simulink model "ddc_model"  (R2023b)
settings: Solver=VariableStepDiscrete  StartTime=0.0  StopTime=DDC_LINEUP_param.endTime  RelTol=1e-3  EnableMultiTasking=on
PreLoadFcn:
  | % Run the setup script when the model is opened
  | setup_ddc_model;
InitFcn:
  | % Run the setup script again just before the
  | % model is run, so that any updates made
  | % after opening are applied.
  | 
  | setup_ddc_model;
StopFcn:
  | ddc_output_analysis;
values from neighbouring files (symbols this model uses):
  DDC_CM_multiplication_factor = 1    [setup_ddc_model.m]
  DDC_CM_NCO1_phase = [0 0 0 0]*2^DDC_LINEUP_param.Complex_NCO1.accum_bit_width    [setup_ddc_model.m]
  DDC_CM_NCO_sync = [0 0 0 0]    [setup_ddc_model.m]
  DDC_CM_number_of_bits_to_shift_left = 0    [setup_ddc_model.m]
undefined symbols (not defined in the file or in its folder): AdvDSPBChannelOutDisplay, COMPLEX_MIXER, DDC_LINEUP_param, dpoly, dspba_ChannelInVis, dspba_ChannelOutVis, dspba_internal_get_channel_ports, evalAionMaskParam, latency, lddc, lddc_lib, mixer_lib, primtype, value
libraries: DSPBAPrim x43, DSPBABase x15, simulink x10, DSPBAFilters x6, DSPBAModelBus x3, DSPBAWaveformSynth x2
(part 2 of 2)

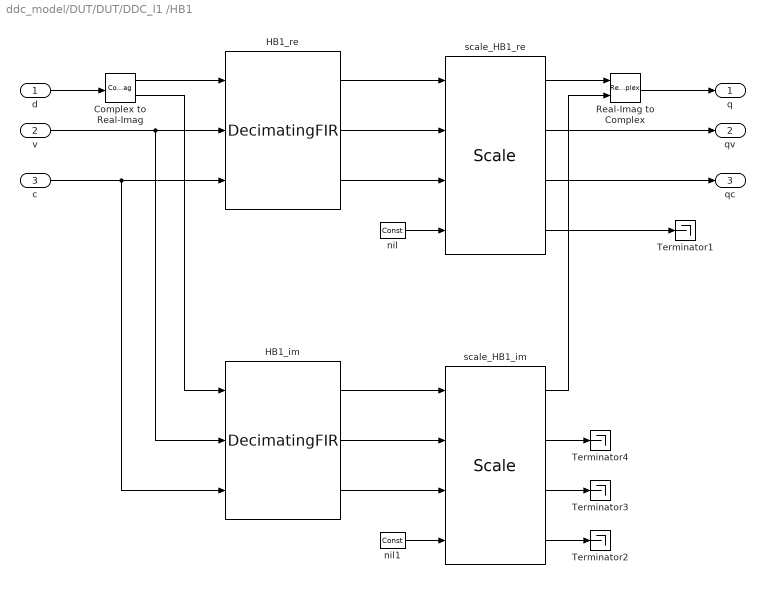
== system ddc_model/DUT/DUT/DDC_l1 /HB1 ==
  d : Inport
  v : Inport  Port=2
  c : Inport  Port=3
  Complex to Real-Imag : ComplexToRealImag
  HB1_im : DSPBAFilters/DecimatingFIR  nInputRate=DDC_LINEUP_param.HB_filt1.SampleRate  decim=DDC_LINEUP_param.HB_filt1.Decimation  nchan=DDC_LINEUP_param.HB_filt1.ChanCount  symmetry=Symmetrical  coef=DDC_LINEUP_param.HB_filt1.coeffs  addr=DDC_LINEUP_param.HB_filter6_3.base_addr  rwmode=Constant  nband=Half Band  exposebus=off  latency=17  version=20090407  recon=off  MM=[0,1,2,3,4,5,6,7,8,9,10,11,12,13,14,15]  resetrezero=off  sharecoef=auto  simulationMode=Standard
  HB1_re : DSPBAFilters/DecimatingFIR  nInputRate=DDC_LINEUP_param.HB_filt1.SampleRate  decim=DDC_LINEUP_param.HB_filt1.Decimation  nchan=DDC_LINEUP_param.HB_filt1.ChanCount  symmetry=Symmetrical  coef=DDC_LINEUP_param.HB_filt1.coeffs  addr=DDC_LINEUP_param.HB_filter6_3.base_addr  rwmode=Constant  nband=Half Band  exposebus=off  latency=17  version=20090407  recon=off  MM=[0,1,2,3,4,5,6,7,8,9,10,11,12,13,14,15]  resetrezero=off  sharecoef=auto  simulationMode=Standard
  Real-Imag to Complex : RealImagToComplex
  Terminator{1..4} (4 alike) : Terminator
  nil : DSPBAPrim/Const  primtype=const  nInputs=0  nOutputs=1  omode=Inherit via internal rule  otype=sfix(16)  scale=2^-15  rndmethod=Unbiased  factor=1  satmethod=Symmetric  shift_vec=[0 1 2 -1]  value=0  inPortNames=['+'; '+';]  outPortNames=[' ']  dspbaimage=dspba_prim.svg  text=fprintf('%s', num2str(value));  style=Optimised  visibilities=8 + 1024  floatPrecision=float32_m23  warnSaturation=on  version=20211007  SampleTime=inf
  nil1 : DSPBAPrim/Const  primtype=const  nInputs=0  nOutputs=1  omode=Inherit via internal rule  otype=sfix(16)  scale=2^-15  rndmethod=Unbiased  factor=1  satmethod=Symmetric  shift_vec=[0 1 2 -1]  value=0  inPortNames=['+'; '+';]  outPortNames=[' ']  dspbaimage=dspba_prim.svg  text=fprintf('%s', num2str(value));  style=Optimised  visibilities=8 + 1024  floatPrecision=float32_m23  warnSaturation=on  version=20211007  SampleTime=inf
  scale_HB1_im : DSPBABase/Scale  otype=sfix(DDC_LINEUP_param.output_word_length)  scale=2^-DDC_LINEUP_param.output_fraction_length  rndmethod=Biased  factor=1  satmethod=None  shift_vec=0  latency=2  simulationMode=Use Global Value  version=20130807
  scale_HB1_re : DSPBABase/Scale  otype=sfix(DDC_LINEUP_param.output_word_length)  scale=2^-DDC_LINEUP_param.output_fraction_length  rndmethod=Biased  factor=1  satmethod=None  shift_vec=0  latency=2  simulationMode=Use Global Value  version=20130807
  q : Outport
  qv : Outport  Port=2
  qc : Outport  Port=3
  wires:
  scale_HB1_re/1 -> Real-Imag to Complex/1
  HB1_re/3 -> scale_HB1_re/3
  c/1 -> HB1_im/3, HB1_re/3
  scale_HB1_re/3 -> qc/1
  scale_HB1_re/2 -> qv/1
  HB1_re/2 -> scale_HB1_re/2
  v/1 -> HB1_im/2, HB1_re/2
  nil1/1 -> scale_HB1_im/4
  scale_HB1_re/4 -> Terminator1/1
  HB1_re/1 -> scale_HB1_re/1
  Complex to Real-Imag/1 -> HB1_re/1
  nil/1 -> scale_HB1_re/4
  d/1 -> Complex to Real-Imag/1
  scale_HB1_im/4 -> Terminator2/1
  HB1_im/1 -> scale_HB1_im/1
  scale_HB1_im/1 -> Real-Imag to Complex/2
  scale_HB1_im/2 -> Terminator4/1
  Complex to Real-Imag/2 -> HB1_im/1
  HB1_im/2 -> scale_HB1_im/2
  scale_HB1_im/3 -> Terminator3/1
  Real-Imag to Complex/1 -> q/1
  HB1_im/3 -> scale_HB1_im/3

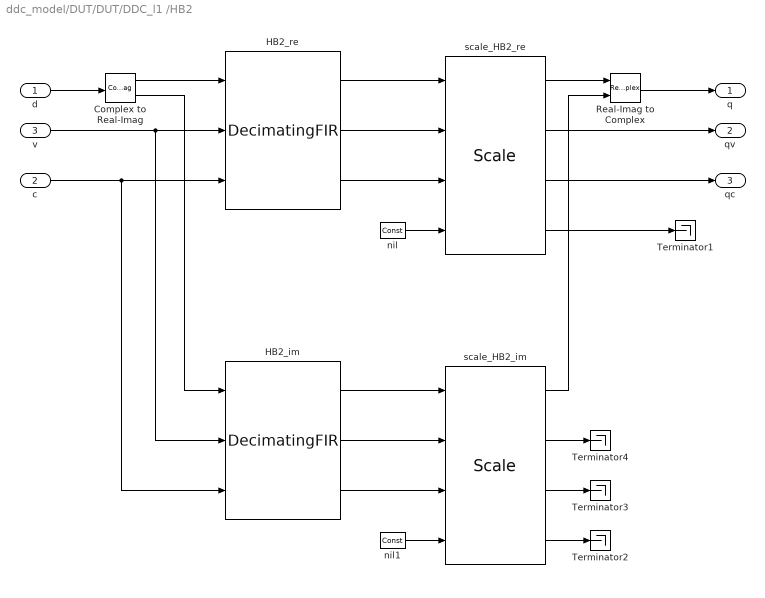
== system ddc_model/DUT/DUT/DDC_l1 /HB2 ==
  d : Inport
  c : Inport  Port=2
  v : Inport  Port=3
  Complex to Real-Imag : ComplexToRealImag
  HB2_im : DSPBAFilters/DecimatingFIR  nInputRate=DDC_LINEUP_param.HB_filt2.SampleRate  decim=DDC_LINEUP_param.HB_filt2.Decimation  nchan=DDC_LINEUP_param.HB_filt2.ChanCount  symmetry=Symmetrical  coef=DDC_LINEUP_param.HB_filt2.coeffs  addr=DDC_LINEUP_param.HB_filter6_3.base_addr  rwmode=Constant  nband=Half Band  exposebus=off  latency=16  version=20090407  recon=off  MM=[0,1,2,3,4,5,6,7,8,9,10,11,12,13,14,15]  resetrezero=off  sharecoef=auto  simulationMode=Standard
  HB2_re : DSPBAFilters/DecimatingFIR  nInputRate=DDC_LINEUP_param.HB_filt2.SampleRate  decim=DDC_LINEUP_param.HB_filt2.Decimation  nchan=DDC_LINEUP_param.HB_filt2.ChanCount  symmetry=Symmetrical  coef=DDC_LINEUP_param.HB_filt2.coeffs  addr=DDC_LINEUP_param.HB_filter6_3.base_addr  rwmode=Constant  nband=Half Band  exposebus=off  latency=16  version=20090407  recon=off  MM=[0,1,2,3,4,5,6,7,8,9,10,11,12,13,14,15]  resetrezero=off  sharecoef=auto  simulationMode=Standard
  Real-Imag to Complex : RealImagToComplex
  Terminator{1..4} (4 alike) : Terminator
  nil : DSPBAPrim/Const  primtype=const  nInputs=0  nOutputs=1  omode=Inherit via internal rule  otype=sfix(16)  scale=2^-15  rndmethod=Unbiased  factor=1  satmethod=Symmetric  shift_vec=[0 1 2 -1]  value=0  inPortNames=['+'; '+';]  outPortNames=[' ']  dspbaimage=dspba_prim.svg  text=fprintf('%s', num2str(value));  style=Optimised  visibilities=8 + 1024  floatPrecision=float32_m23  warnSaturation=on  version=20211007  SampleTime=inf
  nil1 : DSPBAPrim/Const  primtype=const  nInputs=0  nOutputs=1  omode=Inherit via internal rule  otype=sfix(16)  scale=2^-15  rndmethod=Unbiased  factor=1  satmethod=Symmetric  shift_vec=[0 1 2 -1]  value=0  inPortNames=['+'; '+';]  outPortNames=[' ']  dspbaimage=dspba_prim.svg  text=fprintf('%s', num2str(value));  style=Optimised  visibilities=8 + 1024  floatPrecision=float32_m23  warnSaturation=on  version=20211007  SampleTime=inf
  scale_HB2_im : DSPBABase/Scale  otype=sfix(DDC_LINEUP_param.output_word_length)  scale=2^-DDC_LINEUP_param.output_fraction_length  rndmethod=Biased  factor=1  satmethod=None  shift_vec=0  latency=2  simulationMode=Use Global Value  version=20130807
  scale_HB2_re : DSPBABase/Scale  otype=sfix(DDC_LINEUP_param.output_word_length)  scale=2^-DDC_LINEUP_param.output_fraction_length  rndmethod=Biased  factor=1  satmethod=None  shift_vec=0  latency=2  simulationMode=Use Global Value  version=20130807
  q : Outport
  qv : Outport  Port=2
  qc : Outport  Port=3
  wires:
  HB2_im/3 -> scale_HB2_im/3
  Real-Imag to Complex/1 -> q/1
  scale_HB2_im/3 -> Terminator3/1
  HB2_im/2 -> scale_HB2_im/2
  Complex to Real-Imag/2 -> HB2_im/1
  scale_HB2_im/2 -> Terminator4/1
  scale_HB2_im/1 -> Real-Imag to Complex/2
  HB2_im/1 -> scale_HB2_im/1
  scale_HB2_im/4 -> Terminator2/1
  d/1 -> Complex to Real-Imag/1
  nil/1 -> scale_HB2_re/4
  Complex to Real-Imag/1 -> HB2_re/1
  HB2_re/1 -> scale_HB2_re/1
  scale_HB2_re/4 -> Terminator1/1
  nil1/1 -> scale_HB2_im/4
  v/1 -> HB2_im/2, HB2_re/2
  HB2_re/2 -> scale_HB2_re/2
  scale_HB2_re/2 -> qv/1
  scale_HB2_re/3 -> qc/1
  c/1 -> HB2_im/3, HB2_re/3
  HB2_re/3 -> scale_HB2_re/3
  scale_HB2_re/1 -> Real-Imag to Complex/1

== system ddc_model/DUT/DUT/DDC_l1 /routing_reg_hb62hb7 ==
  d : Inport
  dv : Inport  Port=2
  dc : Inport  Port=3
  ChannelIn : DSPBAPrim/ChannelIn  primtype=channelin  nInputs=dspba_internal_get_channel_ports(gcb)  nOutputs=dspba_internal_get_channel_ports(gcb)  omode=Inherit via internal rule  otype=sfix(16)  scale=2^-15  rndmethod=Unbiased  factor=1  satmethod=Symmetric  shift_vec=[0 1 2 -1]  value=1  inPortNames=['v'; 'c'; '0'; '1'; '2'; '3'; '4'; '5'; '6'; '7'; '8'; '9'; 'A'; 'B'; 'D'; 'E'; 'F'; 'G'; 'H'; 'I'; 'J'; 'K'; 'L'; 'M'; 'N'; 'O'; 'P'; 'Q'; 'R'; 'S'; 'T'; 'U'; 'W'; 'X'; 'Y'; 'Z']  outPortNames=['v'; 'c'; '0'; '1'; '2'; '3'; '4'; '5'; '6'; '7'; '8'; '9'; 'A'; 'B'; 'D'; 'E'; 'F'; 'G'; 'H'; 'I'; 'J'; 'K'; 'L'; 'M'; 'N'; 'O'; 'P'; 'Q'; 'R'; 'S'; 'T'; 'U'; 'W'; 'X'; 'Y'; 'Z']  dspbaimage=dspba_prim_channel_tall.svg  text=fprintf('In');  style=Optimised  dataSignals=1  foldingEnabled=off  channels=1  sampleRate=200  packetBeginPresent=off  packetBeginEnabled=off  visibilities=dspba_ChannelInVis(gcb)  scheduleOrigin=on  version=20211214
  ChannelOut : DSPBAPrim/ChannelOut  primtype=channelout  nInputs=dspba_internal_get_channel_ports(gcb)  nOutputs=dspba_internal_get_channel_ports(gcb)  omode=Inherit via internal rule  otype=sfix(16)  scale=2^-15  rndmethod=Unbiased  factor=1  satmethod=Symmetric  shift_vec=[0 1 2 -1]  value=1  inPortNames=['v'; 'c'; '0'; '1'; '2'; '3'; '4'; '5'; '6'; '7'; '8'; '9'; 'A'; 'B'; 'D'; 'E'; 'F'; 'G'; 'H'; 'I'; 'J'; 'K'; 'L'; 'M'; 'N'; 'O'; 'P'; 'Q'; 'R'; 'S'; 'T'; 'U'; 'W'; 'X'; 'Y'; 'Z']  outPortNames=['v'; 'c'; '0'; '1'; '2'; '3'; '4'; '5'; '6'; '7'; '8'; '9'; 'A'; 'B'; 'D'; 'E'; 'F'; 'G'; 'H'; 'I'; 'J'; 'K'; 'L'; 'M'; 'N'; 'O'; 'P'; 'Q'; 'R'; 'S'; 'T'; 'U'; 'W'; 'X'; 'Y'; 'Z']  dspbaimage=dspba_prim_channel_tall.svg  text=fprintf('Out%s', AdvDSPBChannelOutDisplay(latency));  style=Optimised  dataSignals=1  foldingEnabled=off  channels=1  sampleRate=200  packetBeginPresent=off  packetBeginEnabled=off  visibilities=dspba_ChannelOutVis(gcb)  latency=3  version=20211214
  SynthesisInfo : DSPBAPrim/SynthesisInfo  primtype=synthinfo  nInputs=0  nOutputs=0  omode=Inherit via internal rule  otype=sfix(16)  scale=2^-15  rndmethod=Truncate  factor=1  satmethod=Symmetric  shift_vec=[0 1 2 -1]  value=99  inPortNames=[' '; ' ';]  outPortNames=[' ']  dspbaimage=dspba_prim_ctrl.jpg  text=fprintf('Style=%s', style);  style=Scheduled  visibilities=2^17+2^18+2^19+2^20  constraintPair=Channel-In to Channel-Out  constraintRelation=>  constraintLimit=2  modelRefSign=+  modelRef=''  showSchedule=off  simulationMode=Use Global Value  resetMinimization=Conditional - On for ChannelIn/Out only  version=20220106
  q0 : Outport
  qv : Outport  Port=2
  qc : Outport  Port=3
  wires:
  dv/1 -> ChannelIn/1
  d/1 -> ChannelIn/3
  ChannelIn/1 -> ChannelOut/1
  ChannelIn/2 -> ChannelOut/2
  ChannelIn/3 -> ChannelOut/3
  ChannelOut/3 -> q0/1
  ChannelOut/1 -> qv/1
  ChannelOut/2 -> qc/1
  dc/1 -> ChannelIn/2

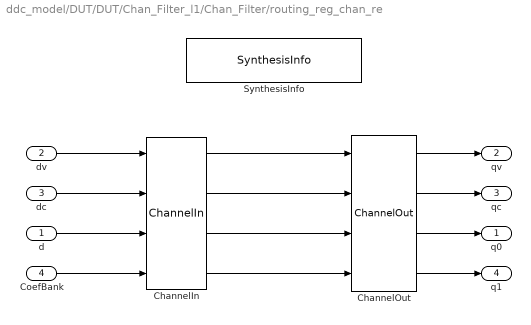
== system ddc_model/DUT/DUT/Chan_Filter_l1/Chan_Filter/routing_reg_chan_re ==
  d : Inport
  dv : Inport  Port=2
  dc : Inport  Port=3
  CoefBank : Inport  Port=4
  ChannelIn : DSPBAPrim/ChannelIn  primtype=channelin  nInputs=dspba_internal_get_channel_ports(gcb)  nOutputs=dspba_internal_get_channel_ports(gcb)  omode=Inherit via internal rule  otype=sfix(16)  scale=2^-15  rndmethod=Unbiased  factor=1  satmethod=Symmetric  shift_vec=[0 1 2 -1]  value=2  inPortNames=['v'; 'c'; '0'; '1'; '2'; '3'; '4'; '5'; '6'; '7'; '8'; '9'; 'A'; 'B'; 'D'; 'E'; 'F'; 'G'; 'H'; 'I'; 'J'; 'K'; 'L'; 'M'; 'N'; 'O'; 'P'; 'Q'; 'R'; 'S'; 'T'; 'U'; 'W'; 'X'; 'Y'; 'Z']  outPortNames=['v'; 'c'; '0'; '1'; '2'; '3'; '4'; '5'; '6'; '7'; '8'; '9'; 'A'; 'B'; 'D'; 'E'; 'F'; 'G'; 'H'; 'I'; 'J'; 'K'; 'L'; 'M'; 'N'; 'O'; 'P'; 'Q'; 'R'; 'S'; 'T'; 'U'; 'W'; 'X'; 'Y'; 'Z']  dspbaimage=dspba_prim_channel_tall.svg  text=fprintf('In');  style=Optimised  dataSignals=2  foldingEnabled=off  channels=1  sampleRate=200  packetBeginPresent=off  packetBeginEnabled=off  visibilities=dspba_ChannelInVis(gcb)  scheduleOrigin=on  version=20211214
  ChannelOut : DSPBAPrim/ChannelOut  primtype=channelout  nInputs=dspba_internal_get_channel_ports(gcb)  nOutputs=dspba_internal_get_channel_ports(gcb)  omode=Inherit via internal rule  otype=sfix(16)  scale=2^-15  rndmethod=Unbiased  factor=1  satmethod=Symmetric  shift_vec=[0 1 2 -1]  value=2  inPortNames=['v'; 'c'; '0'; '1'; '2'; '3'; '4'; '5'; '6'; '7'; '8'; '9'; 'A'; 'B'; 'D'; 'E'; 'F'; 'G'; 'H'; 'I'; 'J'; 'K'; 'L'; 'M'; 'N'; 'O'; 'P'; 'Q'; 'R'; 'S'; 'T'; 'U'; 'W'; 'X'; 'Y'; 'Z']  outPortNames=['v'; 'c'; '0'; '1'; '2'; '3'; '4'; '5'; '6'; '7'; '8'; '9'; 'A'; 'B'; 'D'; 'E'; 'F'; 'G'; 'H'; 'I'; 'J'; 'K'; 'L'; 'M'; 'N'; 'O'; 'P'; 'Q'; 'R'; 'S'; 'T'; 'U'; 'W'; 'X'; 'Y'; 'Z']  dspbaimage=dspba_prim_channel_tall.svg  text=fprintf('Out%s', AdvDSPBChannelOutDisplay(latency));  style=Optimised  dataSignals=2  foldingEnabled=off  channels=1  sampleRate=200  packetBeginPresent=off  packetBeginEnabled=off  visibilities=dspba_ChannelOutVis(gcb)  latency=3  version=20211214
  SynthesisInfo : DSPBAPrim/SynthesisInfo  primtype=synthinfo  nInputs=0  nOutputs=0  omode=Inherit via internal rule  otype=sfix(16)  scale=2^-15  rndmethod=Truncate  factor=1  satmethod=Symmetric  shift_vec=[0 1 2 -1]  value=99  inPortNames=[' '; ' ';]  outPortNames=[' ']  dspbaimage=dspba_prim_ctrl.jpg  text=fprintf('Style=%s', style);  style=Scheduled  visibilities=2^17+2^18+2^19+2^20  constraintPair=Channel-In to Channel-Out  constraintRelation=>  constraintLimit=2  modelRefSign=+  modelRef=''  showSchedule=off  simulationMode=Use Global Value  resetMinimization=Conditional - On for ChannelIn/Out only  version=20220106
  q0 : Outport
  qv : Outport  Port=2
  qc : Outport  Port=3
  q1 : Outport  Port=4
  wires:
  dv/1 -> ChannelIn/1
  d/1 -> ChannelIn/3
  ChannelIn/1 -> ChannelOut/1
  ChannelIn/2 -> ChannelOut/2
  ChannelIn/3 -> ChannelOut/3
  ChannelOut/3 -> q0/1
  ChannelOut/1 -> qv/1
  ChannelOut/2 -> qc/1
  dc/1 -> ChannelIn/2
  ChannelIn/4 -> ChannelOut/4
  CoefBank/1 -> ChannelIn/4
  ChannelOut/4 -> q1/1

== system ddc_model/DUT/DUT/Chan_Filter_l1/Chan_Filter/routing_reg_chan_re1 ==
  d : Inport
  dv : Inport  Port=2
  dc : Inport  Port=3
  CoefBank : Inport  Port=4
  ChannelIn : DSPBAPrim/ChannelIn  primtype=channelin  nInputs=dspba_internal_get_channel_ports(gcb)  nOutputs=dspba_internal_get_channel_ports(gcb)  omode=Inherit via internal rule  otype=sfix(16)  scale=2^-15  rndmethod=Unbiased  factor=1  satmethod=Symmetric  shift_vec=[0 1 2 -1]  value=2  inPortNames=['v'; 'c'; '0'; '1'; '2'; '3'; '4'; '5'; '6'; '7'; '8'; '9'; 'A'; 'B'; 'D'; 'E'; 'F'; 'G'; 'H'; 'I'; 'J'; 'K'; 'L'; 'M'; 'N'; 'O'; 'P'; 'Q'; 'R'; 'S'; 'T'; 'U'; 'W'; 'X'; 'Y'; 'Z']  outPortNames=['v'; 'c'; '0'; '1'; '2'; '3'; '4'; '5'; '6'; '7'; '8'; '9'; 'A'; 'B'; 'D'; 'E'; 'F'; 'G'; 'H'; 'I'; 'J'; 'K'; 'L'; 'M'; 'N'; 'O'; 'P'; 'Q'; 'R'; 'S'; 'T'; 'U'; 'W'; 'X'; 'Y'; 'Z']  dspbaimage=dspba_prim_channel_tall.svg  text=fprintf('In');  style=Optimised  dataSignals=2  foldingEnabled=off  channels=1  sampleRate=200  packetBeginPresent=off  packetBeginEnabled=off  visibilities=dspba_ChannelInVis(gcb)  scheduleOrigin=on  version=20211214
  ChannelOut : DSPBAPrim/ChannelOut  primtype=channelout  nInputs=dspba_internal_get_channel_ports(gcb)  nOutputs=dspba_internal_get_channel_ports(gcb)  omode=Inherit via internal rule  otype=sfix(16)  scale=2^-15  rndmethod=Unbiased  factor=1  satmethod=Symmetric  shift_vec=[0 1 2 -1]  value=2  inPortNames=['v'; 'c'; '0'; '1'; '2'; '3'; '4'; '5'; '6'; '7'; '8'; '9'; 'A'; 'B'; 'D'; 'E'; 'F'; 'G'; 'H'; 'I'; 'J'; 'K'; 'L'; 'M'; 'N'; 'O'; 'P'; 'Q'; 'R'; 'S'; 'T'; 'U'; 'W'; 'X'; 'Y'; 'Z']  outPortNames=['v'; 'c'; '0'; '1'; '2'; '3'; '4'; '5'; '6'; '7'; '8'; '9'; 'A'; 'B'; 'D'; 'E'; 'F'; 'G'; 'H'; 'I'; 'J'; 'K'; 'L'; 'M'; 'N'; 'O'; 'P'; 'Q'; 'R'; 'S'; 'T'; 'U'; 'W'; 'X'; 'Y'; 'Z']  dspbaimage=dspba_prim_channel_tall.svg  text=fprintf('Out%s', AdvDSPBChannelOutDisplay(latency));  style=Optimised  dataSignals=2  foldingEnabled=off  channels=1  sampleRate=200  packetBeginPresent=off  packetBeginEnabled=off  visibilities=dspba_ChannelOutVis(gcb)  latency=3  version=20211214
  SynthesisInfo : DSPBAPrim/SynthesisInfo  primtype=synthinfo  nInputs=0  nOutputs=0  omode=Inherit via internal rule  otype=sfix(16)  scale=2^-15  rndmethod=Truncate  factor=1  satmethod=Symmetric  shift_vec=[0 1 2 -1]  value=99  inPortNames=[' '; ' ';]  outPortNames=[' ']  dspbaimage=dspba_prim_ctrl.jpg  text=fprintf('Style=%s', style);  style=Scheduled  visibilities=2^17+2^18+2^19+2^20  constraintPair=Channel-In to Channel-Out  constraintRelation=>  constraintLimit=2  modelRefSign=+  modelRef=''  showSchedule=off  simulationMode=Use Global Value  resetMinimization=Conditional - On for ChannelIn/Out only  version=20220106
  q0 : Outport
  qv : Outport  Port=2
  qc : Outport  Port=3
  q1 : Outport  Port=4
  wires:
  ChannelOut/4 -> q1/1
  CoefBank/1 -> ChannelIn/4
  ChannelIn/4 -> ChannelOut/4
  dc/1 -> ChannelIn/2
  ChannelOut/2 -> qc/1
  ChannelOut/1 -> qv/1
  ChannelOut/3 -> q0/1
  ChannelIn/3 -> ChannelOut/3
  ChannelIn/2 -> ChannelOut/2
  ChannelIn/1 -> ChannelOut/1
  d/1 -> ChannelIn/3
  dv/1 -> ChannelIn/1
